simulink model "CruiseControl_G_ExecOrderLimCheckSneak_fix"  (R2016a)
settings: Solver=ode3  StartTime=0.0  StopTime=16  FixedStep=0.1  RelTol=1e-3
PreLoadFcn:
  | CruiseControl_dd;
undefined symbols (not defined in the file or in its folder): holdrate, incdec, maxtspeed, mintspeed
settings Model: SnapshotInterval=1  Creator=The MathWorks Inc.  LastModifiedBy=colosky
settings DataIOCC: LimitDataPoints=on  SaveFormat=Array  SaveOutput=off  SaveTime=off
settings OptimizationCC: DefaultParameterBehavior=Inlined  InlineInvariantSignals=on  ExpressionDepthLimit=2147483647  InitFltsAndDblsToZero=on  OptimizeModelRefInitCode=on  LifeSpan=1
settings DebuggingCC: SaveWithParameterizedLinksMsg=none  UnderspecifiedInitializationDetection=Classic  MergeDetectMultiDrivingBlocksExec=none  SolverPrmCheckMsg=warning  FcnCallInpInsideContextMsg=UseLocalSettings  AssertControl=DisableAll  AllowSymbolicDim=off  StateNameClashWarn=warning  StrictBusMsg=ErrorOnBusTreatedAsVector
settings HardwareCC: ProdBitPerPointer=32  ProdLargestAtomicFloat=None  ProdEndianess=Unspecified  ProdWordSize=32  ProdHWDeviceType=32-bit Generic
settings ModelReferenceCC: ModelReferenceNumInstancesAllowed=Single  PropagateSignalLabelsOutOfModel=off
settings SFSimCC: SimParseCustomCode=off
settings RTWCC: SystemTargetFile=ert.tlc  TemplateMakefile=ert_default_tmf  GenerateReport=on  IncludeHyperlinkInReport=on  LaunchReport=on  GenerateTraceInfo=on  GenerateTraceReport=on  GenerateTraceReportSl=on  GenerateTraceReportSf=on  GenerateTraceReportEml=on
settings CodeAppCC: ForceParamTrailComments=on  IgnoreCustomStorageClasses=off  OperatorAnnotations=on  SimulinkDataObjDesc=on  SFDataObjDesc=on  MATLABFcnDesc=on  InsertBlockDesc=on  MATLABSourceComments=on
settings ERTTargetCC: UtilityFuncGeneration=Shared location  GenerateSampleERTMain=on  SupportNonFinite=off  ParenthesesLevel=Maximum  CastingMode=Standards  GenerateSharedConstants=off  InlinedParameterPlacement=NonHierarchical  ERTCustomFileTemplate=example_file_process.tlc  EnableSignedLeftShifts=off  EnableSignedRightShifts=off
settings ConfigComp: CovEnable=on  CovScope=ReferencedModels  CovIncludeTopModel=off  RecordCoverage=on  CovMetricSettings=dcme  CovHtmlReporting=off  CovSaveCumulativeToWorkspaceVar=off  CovSaveSingleToWorkspaceVar=off  CovModelRefEnable=Off  CovSFcnEnable=off  DVMode=PropertyProving  DVMaxProcessTime=3000  DVDisplayUnsatisfiableObjectives=on  DVAutomaticStubbing=off  DVMakeOutputFilesUnique=off  DVParameters=on  DVParametersUseConfig=on  DVModelCoverageObjectives=MCDC  DVMaxTestCaseSteps=500  DVTestSuiteOptimization=CombinedObjectives  DVAssertions=EnableAll  DVProofAssumptions=EnableAll  DVDetectIntegerOverflow=off  DVDetectActiveLogic=on  DVMaxViolationSteps=10  DVSaveDataFile=off  DVReportIncludeGraphics=on  DVDisplayResultsOnModel=on

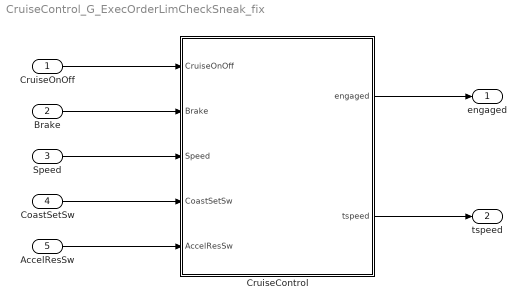
== system CruiseControl_G_ExecOrderLimCheckSneak_fix ==
  CruiseOnOff : Inport  OutDataTypeStr=boolean  PortDimensions=1
  Brake : Inport  Port=2  OutDataTypeStr=boolean  PortDimensions=1
  Speed : Inport  Port=3  OutDataTypeStr=uint8  PortDimensions=1
  CoastSetSw : Inport  Port=4  OutDataTypeStr=boolean  PortDimensions=1
  AccelResSw : Inport  Port=5  OutDataTypeStr=boolean  PortDimensions=1
  CruiseControl : Subsystem  VariantControl=CtrlsVer == CtrlsVerEnum.CtrlG_ExecOrderLimCheckSneak_fix
  engaged : Outport  OutDataTypeStr=boolean  PortDimensions=1
  tspeed : Outport  Port=2  OutDataTypeStr=uint8  PortDimensions=1
  wires:
  CruiseControl/2(tspeed) -> tspeed/1
  CruiseControl/1(engaged) -> engaged/1
  CruiseOnOff/1 -> CruiseControl/1(CruiseOnOff)
  Brake/1 -> CruiseControl/2(Brake)
  Speed/1 -> CruiseControl/3(Speed)
  CoastSetSw/1 -> CruiseControl/4(CoastSetSw)
  AccelResSw/1 -> CruiseControl/5(AccelResSw)

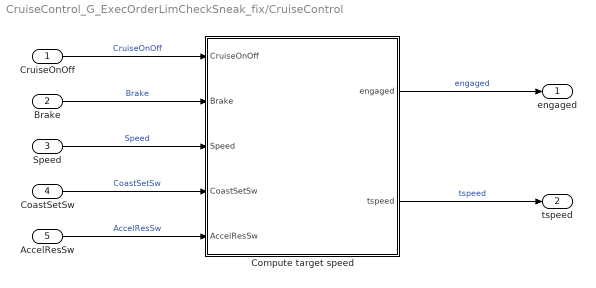
== system CruiseControl_G_ExecOrderLimCheckSneak_fix/CruiseControl ==
  CruiseOnOff : Inport  PortDimensions=1
  Brake : Inport  Port=2  PortDimensions=1
  Speed : Inport  Port=3  PortDimensions=1
  CoastSetSw : Inport  Port=4  PortDimensions=1
  AccelResSw : Inport  Port=5  PortDimensions=1
  Compute target speed : Stateflow chart  TreatAsAtomicUnit=on
  engaged : Outport
  tspeed : Outport  Port=2
  wires:
  Compute target speed/2(tspeed) -> tspeed/1  "tspeed"
  Compute target speed/1(engaged) -> engaged/1  "engaged"
  AccelResSw/1 -> Compute target speed/5(AccelResSw)  "AccelResSw"
  CruiseOnOff/1 -> Compute target speed/1(CruiseOnOff)  "CruiseOnOff"
  Brake/1 -> Compute target speed/2(Brake)  "Brake"
  CoastSetSw/1 -> Compute target speed/4(CoastSetSw)  "CoastSetSw"
  Speed/1 -> Compute target speed/3(Speed)  "Speed"

== stateflow chart CruiseControl_G_ExecOrderLimCheckSneak_fix/CruiseControl/Compute target speed ==
  state OFF
    en:
    engaged = false;
    tspeed = 0;
  state CRUISE
    state ON
      en: engaged = true;
      state Accel
        tspeed = min(tspeed + incdec,maxtspeed);
      state Steady
      state Coast
        tspeed = max(tspeed - incdec,mintspeed);
      (junction 60) -> Accel
      (junction 57) -> (junction 60) : [after(uint32(10)...
          | /holdrate...
          | *incdec,tick)]
      Accel -> (junction 57) [order 2]
      Steady -> Accel [order 1] : [hasChangedTo(AccelResSw,true) ...
          | && tspeed < maxtspeed]
      Accel -> Steady [order 1] : [!AccelResSw ...
          | || tspeed >= maxtspeed]
      (default) -> Steady : {tspeed = Speed;}
      Steady -> Coast [order 2] : [hasChangedTo(CoastSetSw,true) ...
          | && tspeed > mintspeed]
      Coast -> Steady [order 1] : [!CoastSetSw || ...
          | tspeed <= mintspeed]
      (junction 72) -> Coast
      (junction 71) -> (junction 72) : [after(uint32(10) ...
          | /holdrate...
          | *incdec,tick)]
      Coast -> (junction 71) [order 2]
    state STANDBY
      en:
      engaged=false;
    (default) -> STANDBY
    ON -> STANDBY : [Brake||Speed> maxtspeed||Speed<mintspeed]
    STANDBY -> (junction 103) : [~Brake && ...
        | Speed<=maxtspeed && ...
        | Speed>=mintspeed]
    (junction 103) -> Steady [order 1] : [hasChangedTo(AccelResSw,true)...
        | &&tspeed!=0]
    (junction 103) -> (junction 106) [order 2]
    (junction 106) -> ON : [hasChangedTo(CoastSetSw,true)]
  (default) -> OFF
  OFF -> CRUISE : [CruiseOnOff]
  CRUISE -> OFF : [~CruiseOnOff]
  data: engaged output; CruiseOnOff input; Brake input; Speed input; CoastSetSw input; AccelResSw input; tspeed output; incdec parameter; holdrate parameter; maxtspeed parameter; mintspeed parameter
